simulink model "blockdemo"  (Simulink 6.3)
settings: Solver=FixedStepDiscrete  StartTime=0.0  StopTime=10.0  RelTol=1e-3
InitFcn:
  | %% DSPBuilder Start
  | alt_dspbuilder_update_model(bdroot)
  | %% DSPBuilder End
libraries: allblocks_alteradspbuilder2 x5
settings Model: Creator=cpurcell  LastModifiedBy=delphick
settings DebuggingCC: MultiTaskDSMMsg=error

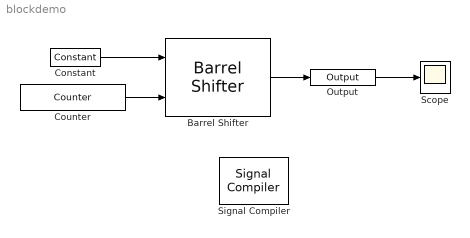
== system blockdemo ==
  Barrel Shifter : allblocks_alteradspbuilder2/Barrel Shifter  BusType=Signed Integer  bwl=8  bwr=8  pipeline=off  ShiftDirection=Shift left  use_aclr=off  UseDedicatedCircuitry=off
  Constant : allblocks_alteradspbuilder2/Constant  mask_cst=-17  BusType=Signed Integer  bwl=8  bwr=0  SpecifyClock=off
  Counter : allblocks_alteradspbuilder2/Counter  BusType=Unsigned Integer  bwl=3  bwr=0  use_modulo=off  modulo=256  SpecifyClock=off  direction=Increment  use_sload=off  use_sset=off  svalue=1  use_ena=off  use_sclr=off
  Output : allblocks_alteradspbuilder2/Output  iofile=C:\workspace_clean\Documentation\DesignExamples\Tutorials\UnitBlocks\Arithmetic\BarrelShifter\tb_blockdemo\blockdemo_Output.capture  BusType=Signed Integer  bwl=8  bwr=0  PORTTYPE=Output
  Scope : Scope
      settings: TimeRange=10  YMin=-130  YMax=130
  Signal Compiler : allblocks_alteradspbuilder2/Signal Compiler  DeviceFamily=Stratix IV  DeviceName=AUTO  EnableSignalTap=off  SignalTapDepth=128  UseBoardBlock=off  StpUseDefaultClock=on  StpClock=clock
  wires:
  Constant/1 -> Barrel Shifter/1
  Counter/1 -> Barrel Shifter/2
  Barrel Shifter/1 -> Output/1
  Output/1 -> Scope/1
